simulink model "malha_fechada_planta"  (R2018b)
settings: Solver=FixedStepAuto  StartTime=0.0  StopTime=10.0  RelTol=1e-3  EnableMultiTasking=on
values from neighbouring files (symbols this model uses):
  dt = 0.001    [Main_Malha_Externa.m]    (also in Main_Malha_Externa_referencia.m; main.m; main_malha_interna.m; otimiza_Dir.m)
  x = fmincon(@otimiza_PIDF,x,[],[],[],[],[0 0 0 0],[inf inf inf inf],@QQQ,options)    [Main_Malha_Externa.m]    (also in Main_Malha_Externa_referencia.m = fmincon(@otimiza_PIDF_referencia,x,[],[],[],[],[0 0 0 0],[in; main.m = fmincon(@otimiza_Esq,x,[],[],[],[],[0 0 0],[inf inf 1400],@Q; main_malha_interna.m = fmincon(@otimiza_Esq,x,[],[],[],[],[0 0 0],[inf inf 1400],@Q; otimiza_Dir.m = X)
undefined symbols (not defined in the file or in its folder): DiscIntNeverNeededParam
settings Model: Creator=exupe  LastModifiedBy=vitor
settings OptimizationCC: LifeSpan=inf
settings DebuggingCC: SFUnexpectedBacktrackingDiag=warning  SFNoUnconditionalDefaultTransitionDiag=warning
settings SFSimCC: SimUseLocalCustomCode=off
settings RTWCC: RTWUseLocalCustomCode=off
settings CodeAppCC: StateflowObjectComments=on
settings GRTTargetCC: TargetLangStandard=C89/C90 (ANSI)  GeneratePreprocessorConditionals=Disable all
settings ConfigComp: CovMetricSettings=dw  CovHtmlReporting=on  CovSaveCumulativeToWorkspaceVar=on  CovSaveSingleToWorkspaceVar=on  CovExternalEMLEnable=off

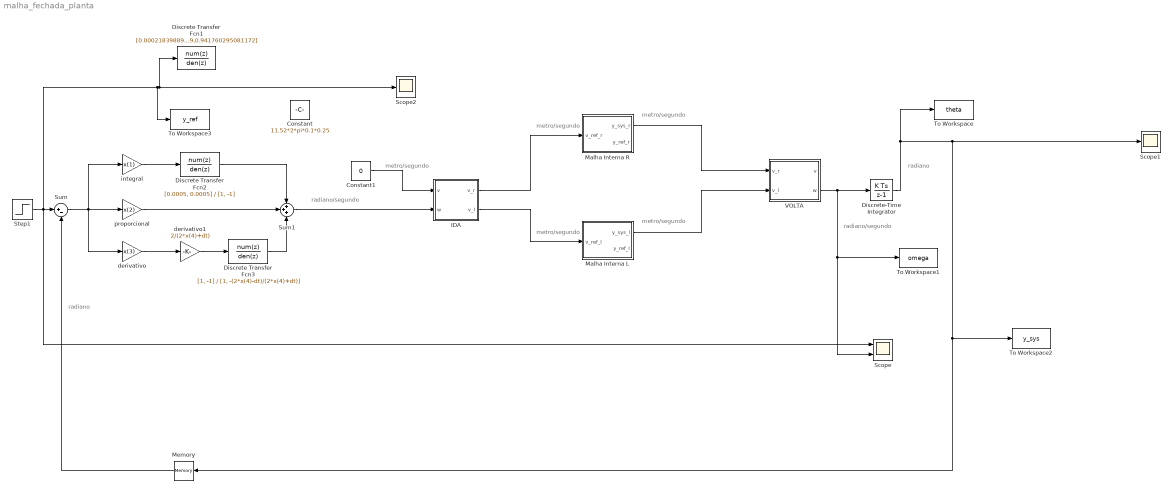
== system malha_fechada_planta ==
  note: radiano
  note: radiano/segundo
  note: metro/segundo
  note: metro/segundo
  note: metro/segundo
  note: metro/segundo
  note: metro/segundo
  note: radiano/segundo
  note: radiano
  Constant : Constant  Value=11.52*2*pi*0.1*0.25
  Constant1 : Constant  Value=0
  Discrete Transfer Fcn1 : DiscreteTransferFcn  Numerator=[0.000218398893445607,0.000436797786891213,0.000218398893445607]  Denominator=[1,-1.94088669950739,0.941760295081172]
  Discrete Transfer Fcn2 : DiscreteTransferFcn  Numerator=[0.0005, 0.0005]  Denominator=[1, -1]
  Discrete Transfer Fcn3 : DiscreteTransferFcn  Numerator=[1, -1]  Denominator=[1, -(2*x(4)-dt)/(2*x(4)+dt)]  SampleTime=0.001
  Discrete-Time Integrator : DiscreteIntegrator  SampleTime=-1  ICPrevOutput=DiscIntNeverNeededParam  ICPrevScaledInput=DiscIntNeverNeededParam
  IDA : Subsystem
  Malha Interna L : Subsystem
  Malha Interna R : Subsystem
  Memory : Memory
  Scope : Scope  NumInputPorts=2
  Scope1 : Scope
  Scope2 : Scope
  Step1 : Step  Time=0  After=0.3  SampleTime=0.001
  Sum : Sum  Inputs=|+-
  Sum1 : Sum  Inputs=+++
  To Workspace : ToWorkspace  VariableName=theta  SaveFormat=Timeseries  SampleTime=-1
  To Workspace1 : ToWorkspace  VariableName=omega  SampleTime=-1
  To Workspace2 : ToWorkspace  VariableName=y_sys  SampleTime=-1
  To Workspace3 : ToWorkspace  VariableName=y_ref  SampleTime=-1
  VOLTA : Subsystem
  derivativo : Gain  Gain=x(3)
  derivativo1 : Gain  Gain=2/(2*x(4)+dt)
  integral : Gain  Gain=x(1)
  proporcional : Gain  Gain=x(2)
  wires:
  IDA/1(v_r) -> Malha Interna R/1(v_ref_r)
  IDA/2(v_l) -> Malha Interna L/1(v_ref_l)
  Malha Interna L/1(y_sys_l) -> VOLTA/2(v_l)
  Malha Interna R/1(y_sys_r) -> VOLTA/1(v_r)
  VOLTA/2(w) -> Discrete-Time Integrator/1, To Workspace1/1, Scope/2
  Sum1/1 -> IDA/2(w)
  Constant1/1 -> IDA/1(v)
  Step1/1 -> Scope/1, To Workspace3/1, Scope2/1, Discrete Transfer Fcn1/1, Sum/1
  Discrete Transfer Fcn2/1 -> Sum1/1
  integral/1 -> Discrete Transfer Fcn2/1
  Memory/1 -> Sum/2
  proporcional/1 -> Sum1/2
  Discrete Transfer Fcn3/1 -> Sum1/3
  Sum/1 -> derivativo/1, integral/1, proporcional/1
  derivativo/1 -> derivativo1/1
  derivativo1/1 -> Discrete Transfer Fcn3/1
  Discrete-Time Integrator/1 -> To Workspace/1, Scope1/1, To Workspace2/1, Memory/1

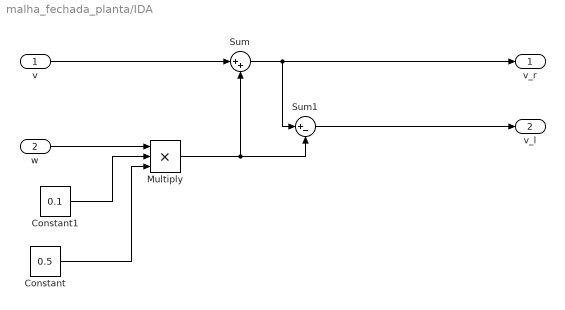
== system malha_fechada_planta/IDA ==
  v : Inport
  w : Inport  Port=2
  Constant : Constant  Value=0.5
  Constant1 : Constant  Value=0.1
  Multiply : Product  Inputs=3
  Sum : Sum  Inputs=|++
  Sum1 : Sum  Inputs=|+-
  v_r : Outport
  v_l : Outport  Port=2
  wires:
  Multiply/1 -> Sum1/2, Sum/2
  Sum1/1 -> v_l/1
  Constant1/1 -> Multiply/2
  v/1 -> Sum/1
  w/1 -> Multiply/1
  Sum/1 -> v_r/1, Sum1/1
  Constant/1 -> Multiply/3

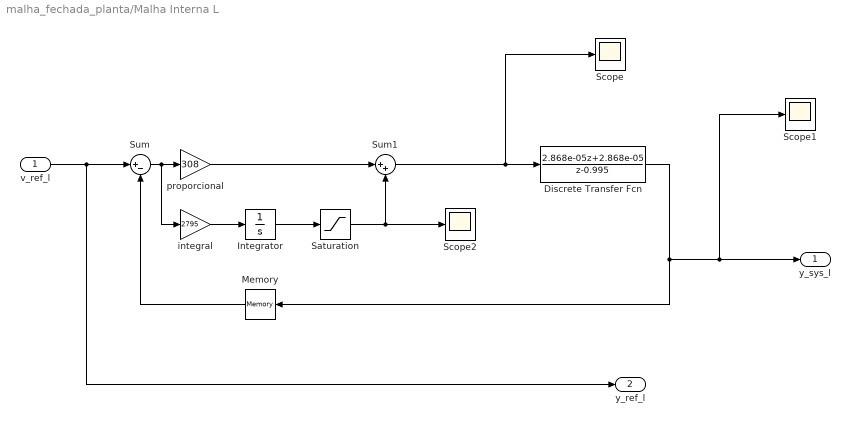
== system malha_fechada_planta/Malha Interna L ==
  v_ref_l : Inport
  Discrete Transfer Fcn : DiscreteTransferFcn  Numerator=[2.868e-05 2.868e-05]  Denominator=[1 -0.995]  SampleTime=0.001
  Integrator : Integrator
  Memory : Memory
  Saturation : Saturate  UpperLimit=1232  LowerLimit=0
  Scope : Scope
  Scope1 : Scope
  Scope2 : Scope
  Sum : Sum  Inputs=|+-
  Sum1 : Sum  Inputs=|++
  integral : Gain  Gain=2795
  proporcional : Gain  Gain=308
  y_sys_l : Outport
  "y_ref_l " : Outport  Port=2
  wires:
  Memory/1 -> Sum/2
  Saturation/1 -> Scope2/1, Sum1/2
  proporcional/1 -> Sum1/1
  v_ref_l/1 -> "y_ref_l "/1, Sum/1
  Sum1/1 -> Scope/1, Discrete Transfer Fcn/1
  Discrete Transfer Fcn/1 -> Memory/1, y_sys_l/1, Scope1/1
  integral/1 -> Integrator/1
  Sum/1 -> integral/1, proporcional/1
  Integrator/1 -> Saturation/1

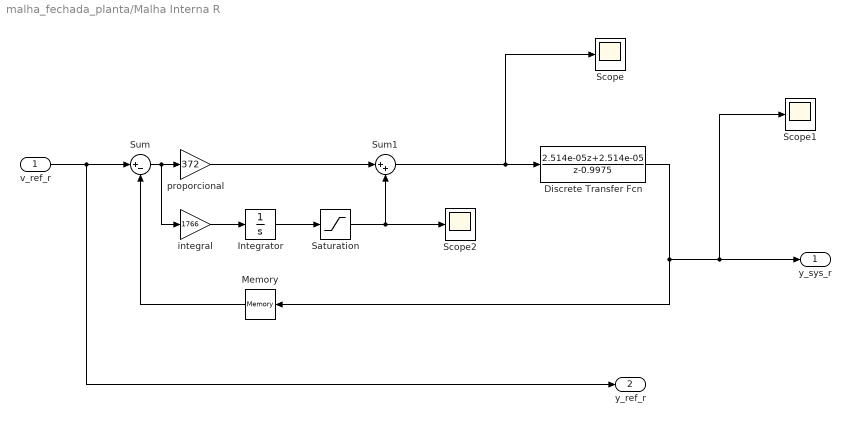
== system malha_fechada_planta/Malha Interna R ==
  v_ref_r : Inport
  Discrete Transfer Fcn : DiscreteTransferFcn  Numerator=[2.514e-05 2.514e-05]  Denominator=[1 -0.9975]  SampleTime=0.001
  Integrator : Integrator
  Memory : Memory
  Saturation : Saturate  UpperLimit=1000  LowerLimit=0
  Scope : Scope
  Scope1 : Scope
  Scope2 : Scope
  Sum : Sum  Inputs=|+-
  Sum1 : Sum  Inputs=|++
  integral : Gain  Gain=1766
  proporcional : Gain  Gain=372
  y_sys_r : Outport
  "y_ref_r " : Outport  Port=2
  wires:
  Memory/1 -> Sum/2
  Saturation/1 -> Scope2/1, Sum1/2
  proporcional/1 -> Sum1/1
  v_ref_r/1 -> "y_ref_r "/1, Sum/1
  Sum1/1 -> Scope/1, Discrete Transfer Fcn/1
  Discrete Transfer Fcn/1 -> Memory/1, y_sys_r/1, Scope1/1
  integral/1 -> Integrator/1
  Sum/1 -> integral/1, proporcional/1
  Integrator/1 -> Saturation/1

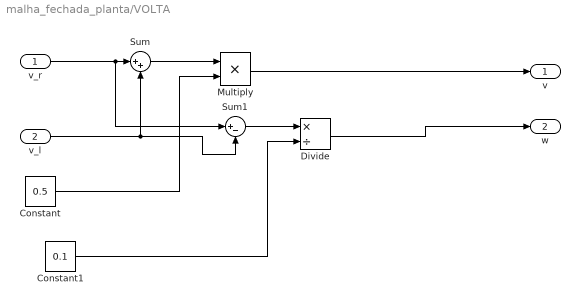
== system malha_fechada_planta/VOLTA ==
  v_r : Inport
  v_l : Inport  Port=2
  Constant : Constant  Value=0.5
  Constant1 : Constant  Value=0.1
  Divide : Product  Inputs=*/
  Multiply : Product
  Sum : Sum  Inputs=|++
  Sum1 : Sum  Inputs=|+-
  v : Outport
  w : Outport  Port=2
  wires:
  Sum/1 -> Multiply/1
  v_l/1 -> Sum1/2, Sum/2
  Sum1/1 -> Divide/1
  v_r/1 -> Sum1/1, Sum/1
  Constant1/1 -> Divide/2
  Multiply/1 -> v/1
  Divide/1 -> w/1
  Constant/1 -> Multiply/2
